simulink model "model"  (R2016a)
settings: Solver=FixedStepDiscrete  SolverMode=SingleTasking  StartTime=0.0  StopTime=10.0  RelTol=1e-3
values from neighbouring files (symbols this model uses):
  Alpha = 0.08737    [constantes.m]
  Ca_CIC = 10    [constantes.m]
  Ce = 0.08737    [constantes.m]
  Cm = 10    [constantes.m]
  Fp_Corr_factor1 = 1    [constantes.m]
  FTS_a = 1    [constantes.m]
  FTS_b = 0.005    [constantes.m]
  K2_CIC = 1    [constantes.m]
  R_FTS = 10    [constantes.m]
  teta_Ad = -0.001416665    [constantes.m]
  teta_Bd = 2.11    [constantes.m]
settings Model: Creator=HP  LastModifiedBy=HP
settings OptimizationCC: DefaultParameterBehavior=Inlined  UseDivisionForNetSlopeComputation=on  UseFloatMulNetSlope=on  InlineInvariantSignals=on  PassReuseOutputArgsAs=Individual arguments  ZeroExternalMemoryAtStartup=off  ZeroInternalMemoryAtStartup=off  NoFixptDivByZeroProtection=on  EfficientFloat2IntCast=on  OptimizeModelRefInitCode=on  LifeSpan=1
settings HardwareCC: ProdBitPerPointer=32  ProdWordSize=32  ProdHWDeviceType=Intel->x86-32 (Windows32)
settings RTWCC: SystemTargetFile=ert.tlc  TemplateMakefile=ert_default_tmf  GenerateReport=on  IncludeHyperlinkInReport=on  LaunchReport=on  GenerateTraceInfo=on  GenerateTraceReport=on  GenerateTraceReportSl=on  GenerateTraceReportSf=on  GenerateTraceReportEml=on  GenerateCodeMetricsReport=on
settings CodeAppCC: ForceParamTrailComments=on  IgnoreCustomStorageClasses=off  OperatorAnnotations=on  SimulinkDataObjDesc=on  SFDataObjDesc=on  MATLABFcnDesc=on  CustomSymbolStrGlobalVar=rt$N$M  CustomSymbolStrType=$N$M  CustomSymbolStrFcn=$N$M$F  CustomSymbolStrMacro=$N$M  InsertBlockDesc=on  MATLABSourceComments=on
settings ERTTargetCC: GenerateSampleERTMain=on  IncludeMdlTerminateFcn=off  CombineSignalStateStructs=on  SupportAbsoluteTime=off  SupportComplex=off  SupportNonInlinedSFcns=on  InlinedParameterPlacement=NonHierarchical  ERTCustomFileTemplate=example_file_process.tlc  ERTFilePackagingFormat=CompactWithDataFile

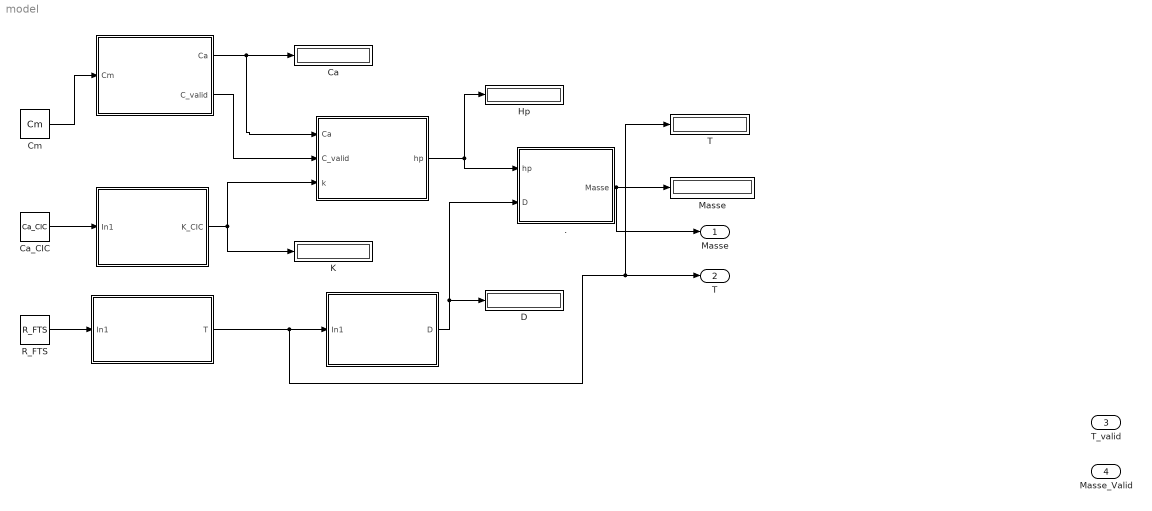
== system model ==
  " " : Subsystem
  "  " : Subsystem
  "   " : Subsystem
  "    " : Subsystem
  "      " : Subsystem
  "         Masse " : Display
  "   Ca" : Display
  "   D" : Display
  "   Hp" : Display
  "   K" : Display
  "   T         " : Display
  . : MATLAB Function  TreatAsAtomicUnit=on
  Ca_CIC : Constant  Value=Ca_CIC
  Cm : Constant  Value=Cm
  R_FTS : Constant  Value=R_FTS
  Masse : Outport
  T : Outport  Port=2
  T_valid : Outport  Port=3
  Masse_Valid : Outport  Port=4
  wires:
  ./1(Masse) -> Masse/1, "         Masse "/1
  "    "/1(hp) -> ./1(hp), "   Hp"/1
  Cm/1 -> " "/1(Cm)
  " "/1(Ca) -> "    "/1(Ca), "   Ca"/1
  " "/2(C_valid) -> "    "/2(C_valid)
  Ca_CIC/1 -> "  "/1(In1)
  "  "/1(K_CIC) -> "   K"/1, "    "/3(k)
  "   "/1(T) -> T/1, "   T         "/1, "      "/1(In1)
  R_FTS/1 -> "   "/1(In1)
  "      "/1(D) -> "   D"/1, ./2(D)

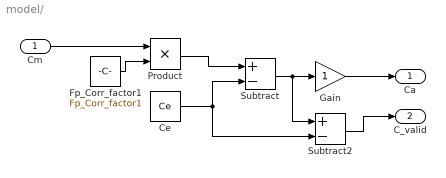
== system model/  ==
  Cm : Inport
  Ce : Constant  Value=Ce
  Fp_Corr_factor1 : Constant  Value=Fp_Corr_factor1
  Gain : Gain
  Product : Product
  Subtract : Sum  Inputs=+-
  Subtract2 : Sum  Inputs=+-
  Ca : Outport
  C_valid : Outport  Port=2
  wires:
  Fp_Corr_factor1/1 -> Product/2
  Product/1 -> Subtract/1
  Cm/1 -> Product/1
  Subtract/1 -> Gain/1, Subtract2/1
  Ce/1 -> Subtract2/2, Subtract/2
  Gain/1 -> Ca/1
  Subtract2/1 -> C_valid/1

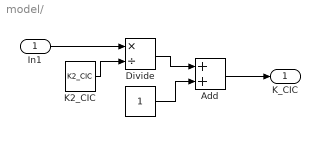
== system model/   ==
  In1 : Inport
  "    " : Constant
  Add : Sum
  Divide : Product  Inputs=*/
  K2_CIC : Constant  Value=K2_CIC
  K_CIC : Outport
  wires:
  K2_CIC/1 -> Divide/2
  In1/1 -> Divide/1
  "    "/1 -> Add/2
  Divide/1 -> Add/1
  Add/1 -> K_CIC/1

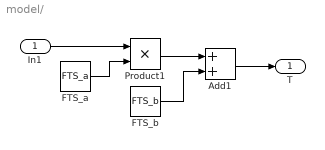
== system model/    ==
  In1 : Inport
  Add1 : Sum
  FTS_a : Constant  Value=FTS_a
  FTS_b : Constant  Value=FTS_b
  Product1 : Product
  T : Outport
  wires:
  In1/1 -> Product1/1
  Add1/1 -> T/1
  Product1/1 -> Add1/1
  FTS_a/1 -> Product1/2
  FTS_b/1 -> Add1/2

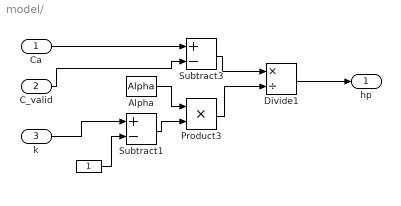
== system model/     ==
  Ca : Inport
  C_valid : Inport  Port=2
  k : Inport  Port=3
  "      " : Constant
  Alpha : Constant  Value=Alpha
  Divide1 : Product  Inputs=*/
  Product3 : Product
  Subtract1 : Sum  Inputs=+-
  Subtract3 : Sum  Inputs=+-
  hp : Outport
  wires:
  "      "/1 -> Subtract1/2
  Ca/1 -> Subtract3/1
  k/1 -> Subtract1/1
  Alpha/1 -> Product3/1
  Product3/1 -> Divide1/2
  C_valid/1 -> Subtract3/2
  Subtract3/1 -> Divide1/1
  Divide1/1 -> hp/1
  Subtract1/1 -> Product3/2

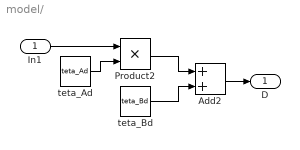
== system model/       ==
  In1 : Inport
  Add2 : Sum
  Product2 : Product
  teta_Ad : Constant  Value=teta_Ad
  teta_Bd : Constant  Value=teta_Bd
  D : Outport
  wires:
  In1/1 -> Product2/1
  teta_Bd/1 -> Add2/2
  teta_Ad/1 -> Product2/2
  Product2/1 -> Add2/1
  Add2/1 -> D/1

== matlab function model/. ==
  data: hp input; Masse output; D input
function Masse = fcn(hp,D)
%#les Ai sont des choix arbitraires
A0 = 0;
A1 = 1;
A2 = 2;
A3 = 0.5;
A4 = 0.05;
A5 = 1;
A6 = 1.5;
Mt_corr_slop = 1;
Mt_corr_offset = 0;
Vtunususable = 72.41 ;
volume = A0 + A1*hp + A2*hp^2 +  A3*hp^3 + A4*hp^4 + A5*hp^5 + A6*hp^6;
Masse =(volume- Vtunususable) * D * Mt_corr_slop + Mt_corr_offset;
end
